simulink model "doubling"  (R2025b)
settings: Solver=FixedStepDiscrete  StartTime=0.0  StopTime=inf  RelTol=1e-3  EnableMultiTasking=on
model workspace (MAT data in the model file):
  Bypass = 0
  Delay_ms = 50
  Depth = 0.5
  Spread = 0
settings Model: Creator=linogarciamorales  LastModifiedBy=linogarciamorales
settings SolverCC: PositivePriorityOrder=on
settings OptimizationCC: EnhancedBackFolding=on  PassReuseOutputArgsAs=Individual arguments  ZeroExternalMemoryAtStartup=off  ZeroInternalMemoryAtStartup=off  MaxStackSize=200000  OptimizeBlockOrder=speed  DifferentSizesBufferReuse=on  OptimizationCustomize=off  EfficientTunableParamExpr=on
settings DebuggingCC: ParameterTunabilityLossMsg=error
settings HardwareCC: ProdBitPerLong=64.0  ProdLargestAtomicInteger=LongLong  ProdLargestAtomicFloat=Double  ProdLongLongMode=on  ProdHWDeviceType=ARM Compatible->ARM Cortex-A (64-bit)
settings RTWCC: SystemTargetFile=ert.tlc  HardwareBoard=Raspberry Pi (64bit)  TLCOptions="-aInlineSetEventsForThisBaseRateFcn=TLC_FALSE -aSuppressMultiTaskScheduler=TLC_FALSE  -aRateBasedStepFcn=0"  GenCodeOnly=on  TemplateMakefile=ert_default_tmf  BuildConfiguration=Faster Runs  PortableWordSizes=on  Description=Embedded Coder
settings CodeAppCC: ForceParamTrailComments=on  IgnoreCustomStorageClasses=off  OperatorAnnotations=on  SimulinkDataObjDesc=on  SFDataObjDesc=on  InsertBlockDesc=on
settings ERTTargetCC: ExtModeTransport=2.0  ExtModeStaticAlloc=on  ExtModeMexFile=ext_xcp  ExtModeIntrfLevel=Level2 - Open  InlinedParameterPlacement=Hierarchical  CodeReplacementLibrary=ARM Cortex-A CMSIS  SupportNonInlinedSFcns=on  SupportVariableSizeSignals=on

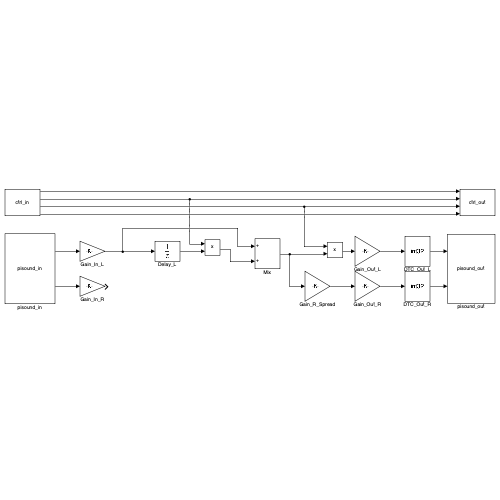
[thumbnail: Simulink's stored preview of the top-level diagram]
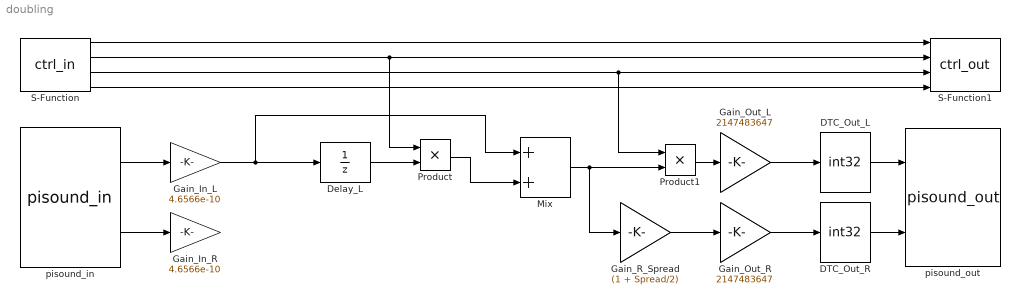
== system doubling ==
  DTC_Out_L : DataTypeConversion  OutDataTypeStr=int32  SaturateOnIntegerOverflow=off  RndMeth=Floor
  DTC_Out_R : DataTypeConversion  OutDataTypeStr=int32  SaturateOnIntegerOverflow=off  RndMeth=Floor
  Delay_L : UnitDelay  SampleTime=-1  HasFrameUpgradeWarning=on
  Gain_In_L : Gain  Gain=4.6566e-10  OutDataTypeStr=double
  Gain_In_R : Gain  Gain=4.6566e-10  OutDataTypeStr=double
  Gain_Out_L : Gain  Gain=2147483647
  Gain_Out_R : Gain  Gain=2147483647
  Gain_R_Spread : Gain  Gain=(1 + Spread/2)
  Mix : Sum
  Product : Product
  Product1 : Product
  S-Function : S-Function  FunctionName=ctrl_in  Parameters=48000, 128, 4  SFunctionDeploymentMode=off  EnableBusSupport=off
  S-Function1 : S-Function  FunctionName=ctrl_out  Parameters=48000, 128, 4  SFunctionDeploymentMode=off  EnableBusSupport=off
  pisound_in : S-Function  FunctionName=pisound_in  Parameters=48000, 128, 0  SFunctionDeploymentMode=off  EnableBusSupport=off
  pisound_out : S-Function  FunctionName=pisound_out  Parameters=48000, 128, 0  SFunctionDeploymentMode=off  EnableBusSupport=off
  wires:
  pisound_in/1 -> Gain_In_L/1
  pisound_in/2 -> Gain_In_R/1
  Gain_In_L/1 -> Delay_L/1, Mix/1
  Delay_L/1 -> Product/2
  Product/1 -> Mix/2
  Mix/1 -> Gain_R_Spread/1, Product1/2
  Product1/1 -> Gain_Out_L/1
  Gain_R_Spread/1 -> Gain_Out_R/1
  Gain_Out_L/1 -> DTC_Out_L/1
  Gain_Out_R/1 -> DTC_Out_R/1
  DTC_Out_L/1 -> pisound_out/1
  DTC_Out_R/1 -> pisound_out/2
  S-Function/2 -> Product/1, S-Function1/2
  S-Function/3 -> S-Function1/3, Product1/1
  S-Function/1 -> S-Function1/1
  S-Function/4 -> S-Function1/4
